simulink model "simulacion_tanques"  (R2018a)
settings: Solver=FixedStepAuto  StartTime=0.0  StopTime=4000  FixedStep=1  RelTol=1e-3
InitFcn:
  | parametros
values from neighbouring files (symbols this model uses):
  A = [A11 A12 A13 ; A21 A22 A23 ; A31 A32 A33 ]    [parametros.m]
  B = [B11 B12 ; B21 B22 ;B31 B32 ]    [parametros.m]
  C = eye(3)    [parametros.m]
  flow_rate_1_ptf = 0.35e-4    (= 3.5e-05)    [ini_para.m]    (also in parametros.m)
  flow_rate_2_ptf = 0.375e-4    (= 3.75e-05)    [ini_para.m]    (also in parametros.m)
  h_max = 0.62    [ini_para.m]    (also in parametros.m)
  h_min = 0    [ini_para.m]    (also in parametros.m)
  K1 = [21.6 3 -5;2.9 19 -4]*10e-4    [ini_para.m]    (also in parametros.m; uio_linear.m = K1')
  K2 = [-0.95 -0.32;-0.3 -0.91]*10e-4    [ini_para.m]    (also in parametros.m)
  level_1_ini = 0.4    [ini_para.m]    (also in parametros.m)
  level_1_ptf = 0.4    [ini_para.m]    (also in parametros.m)
  level_2_ini = 0.2    [ini_para.m]    (also in parametros.m)
  level_2_ptf = 0.2    [ini_para.m]    (also in parametros.m)
  level_3_ini = 0.3    [ini_para.m]    (also in parametros.m)
  level_3_ptf = 0.3    [ini_para.m]    (also in parametros.m)
  q_max = 1.5e-4    (= 0.00015)    [ini_para.m]    (also in parametros.m)
  q_min = 0    [ini_para.m]    (also in parametros.m)
  Te = 1    [ini_para.m]    (also in parametros.m)
undefined symbols (not defined in the file or in its folder): DiscIntNeverNeededParam
settings Model: Creator=cmparedes  LastModifiedBy=cmparedes

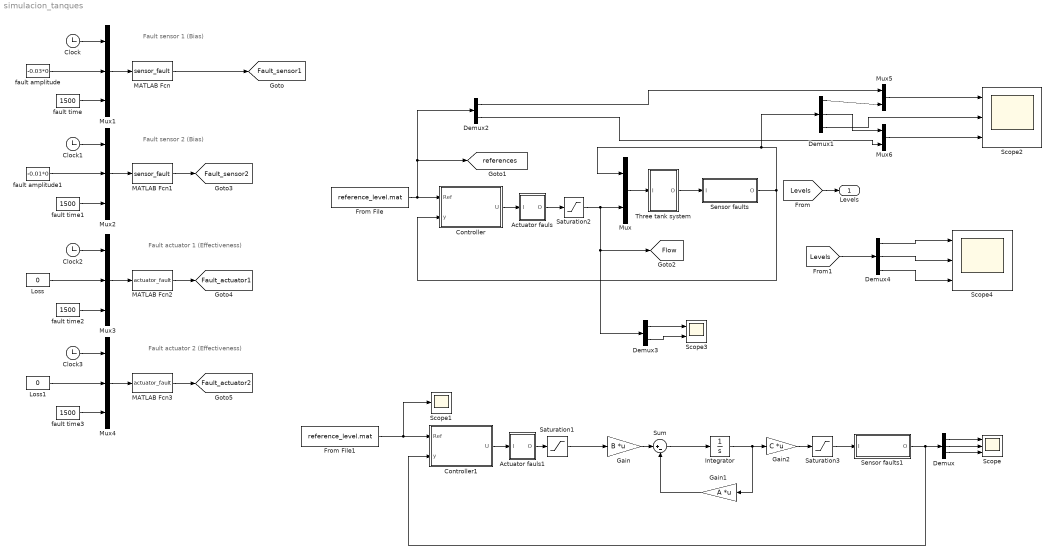
== system simulacion_tanques ==
  note: Fault actuator 2 (Effectiveness)
  note: Fault actuator 1 (Effectiveness)
  note: Fault sensor 1 (Bias)
  note: Fault sensor 2 (Bias)
  Actuator fauls : Subsystem
  Actuator fauls1 : Subsystem
  Clock{,1..3} (4 alike) : Clock
  Controller : Subsystem
  Controller1 : Subsystem
  Demux : Demux  Outputs=3
  Demux1 : Demux  Outputs=3
  Demux2 : Demux  Outputs=2
  Demux3 : Demux  Outputs=2
  Demux4 : Demux  Outputs=3
  From File : FromFile  FileName=reference_level.mat  SampleTime=1
  From File1 : FromFile  FileName=reference_level.mat  SampleTime=1
  Gain : Gain  Gain=B  Multiplication=Matrix(K*u)
  Gain1 : Gain  Gain=A  Multiplication=Matrix(K*u)
  Gain2 : Gain  Gain=C  Multiplication=Matrix(K*u)
  Integrator : Integrator  InitialCondition=[level_1_ini;level_3_ini;level_2_ini]
  Loss : Constant  Value=0
  Loss1 : Constant  Value=0
  MATLAB Fcn : MATLABFcn  MATLABFcn=sensor_fault
  MATLAB Fcn1 : MATLABFcn  MATLABFcn=sensor_fault
  MATLAB Fcn2 : MATLABFcn  MATLABFcn=actuator_fault
  MATLAB Fcn3 : MATLABFcn  MATLABFcn=actuator_fault
  Mux : Mux  Inputs=2
  Mux{1..4} (4 alike) : Mux  Inputs=3
  Mux5 : Mux  Inputs=2
  Mux6 : Mux  Inputs=2
  Saturation1 : Saturate  UpperLimit=q_max  LowerLimit=q_min
  Saturation2 : Saturate  UpperLimit=q_max  LowerLimit=q_min
  Saturation3 : Saturate  UpperLimit=h_max  LowerLimit=h_min
  Scope : Scope  NumInputPorts=3
  Scope1 : Scope
  Scope2 : Scope  NumInputPorts=3
  Scope3 : Scope  NumInputPorts=2
  Scope4 : Scope  NumInputPorts=3
  Sensor faults : Subsystem
  Sensor faults1 : Subsystem
  Sum : Sum  Inputs=|+-
  Three tank system : Subsystem
  fault amplitude : Constant  Value=-0.03*0
  fault amplitude1 : Constant  Value=-0.01*0
  fault time{,1..3} (4 alike) : Constant  Value=1500
  Levels : Outport
  tag scope: Fault_actuator1=global, Fault_actuator2=global, Fault_sensor1=global, Fault_sensor2=global, Flow=global, references=global
  wires:
  Three tank system/1(O) -> Sensor faults/1(I)
  [Levels] -> Levels/1
  Actuator fauls/1(O) -> Saturation2/1
  Sensor faults/1(O) -> Demux1/1, Mux/1, Controller/2(y)
  Saturation2/1 -> Mux/2, Demux3/1, [Flow]
  From File/1 -> Demux2/1, [references], Controller/1(Ref)
  Mux/1 -> Three tank system/1(I)
  Controller/1(U) -> Actuator fauls/1(I)
  Clock1/1 -> Mux2/1
  fault time1/1 -> Mux2/3
  Loss1/1 -> Mux4/2
  Clock/1 -> Mux1/1
  MATLAB Fcn3/1 -> [Fault_actuator2]
  fault time3/1 -> Mux4/3
  MATLAB Fcn2/1 -> [Fault_actuator1]
  Mux3/1 -> MATLAB Fcn2/1
  Clock3/1 -> Mux4/1
  fault amplitude/1 -> Mux1/2
  Mux2/1 -> MATLAB Fcn1/1
  MATLAB Fcn/1 -> [Fault_sensor1]
  Loss/1 -> Mux3/2
  MATLAB Fcn1/1 -> [Fault_sensor2]
  fault time/1 -> Mux1/3
  fault time2/1 -> Mux3/3
  Mux1/1 -> MATLAB Fcn/1
  Clock2/1 -> Mux3/1
  Mux4/1 -> MATLAB Fcn3/1
  fault amplitude1/1 -> Mux2/2
  Gain/1 -> Sum/1
  Sum/1 -> Integrator/1
  Gain1/1 -> Sum/2
  Integrator/1 -> Gain2/1, Gain1/1
  Gain2/1 -> Saturation3/1
  Sensor faults1/1(O) -> Demux/1, Controller1/2(y)
  Actuator fauls1/1(O) -> Saturation1/1
  Controller1/1(U) -> Actuator fauls1/1(I)
  Saturation1/1 -> Gain/1
  From File1/1 -> Scope1/1, Controller1/1(Ref)
  Saturation3/1 -> Sensor faults1/1(I)
  Demux/1 -> Scope/1
  Demux/2 -> Scope/2
  Demux/3 -> Scope/3
  Demux1/1 -> Mux5/2
  Demux2/1 -> Mux5/1
  Mux5/1 -> Scope2/1
  Demux2/2 -> Mux6/2
  Mux6/1 -> Scope2/3
  Demux1/2 -> Mux6/1
  Demux1/3 -> Scope2/2
  Demux3/1 -> Scope3/1
  Demux3/2 -> Scope3/2
  [Levels] -> Demux4/1
  Demux4/1 -> Scope4/1
  Demux4/2 -> Scope4/2
  Demux4/3 -> Scope4/3

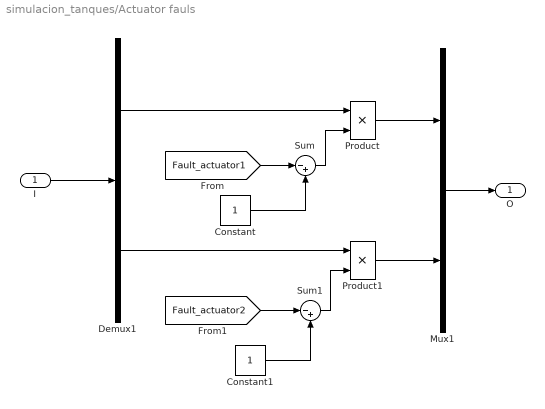
== system simulacion_tanques/Actuator fauls ==
  I : Inport
  Constant : Constant
  Constant1 : Constant
  Demux1 : Demux  Outputs=2
  Mux1 : Mux  Inputs=2
  Product : Product  SaturateOnIntegerOverflow=on  OutDataTypeStr=Inherit: Same as first input
  Product1 : Product  SaturateOnIntegerOverflow=on  OutDataTypeStr=Inherit: Same as first input
  Sum : Sum  Inputs=|-+  SaturateOnIntegerOverflow=on
  Sum1 : Sum  Inputs=|-+  SaturateOnIntegerOverflow=on
  O : Outport
  wires:
  Product1/1 -> Mux1/2
  Demux1/2 -> Product1/1
  Product/1 -> Mux1/1
  Demux1/1 -> Product/1
  Mux1/1 -> O/1
  I/1 -> Demux1/1
  [Fault_actuator1] -> Sum/1
  Constant/1 -> Sum/2
  Sum/1 -> Product/2
  [Fault_actuator2] -> Sum1/1
  Sum1/1 -> Product1/2
  Constant1/1 -> Sum1/2

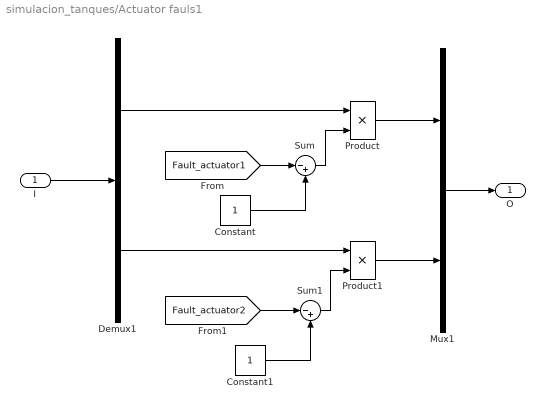
== system simulacion_tanques/Actuator fauls1 ==
  I : Inport
  Constant : Constant
  Constant1 : Constant
  Demux1 : Demux  Outputs=2
  Mux1 : Mux  Inputs=2
  Product : Product  SaturateOnIntegerOverflow=on  OutDataTypeStr=Inherit: Same as first input
  Product1 : Product  SaturateOnIntegerOverflow=on  OutDataTypeStr=Inherit: Same as first input
  Sum : Sum  Inputs=|-+  SaturateOnIntegerOverflow=on
  Sum1 : Sum  Inputs=|-+  SaturateOnIntegerOverflow=on
  O : Outport
  wires:
  Product1/1 -> Mux1/2
  Demux1/2 -> Product1/1
  Product/1 -> Mux1/1
  Demux1/1 -> Product/1
  Mux1/1 -> O/1
  I/1 -> Demux1/1
  [Fault_actuator1] -> Sum/1
  Constant/1 -> Sum/2
  Sum/1 -> Product/2
  [Fault_actuator2] -> Sum1/1
  Sum1/1 -> Product1/2
  Constant1/1 -> Sum1/2

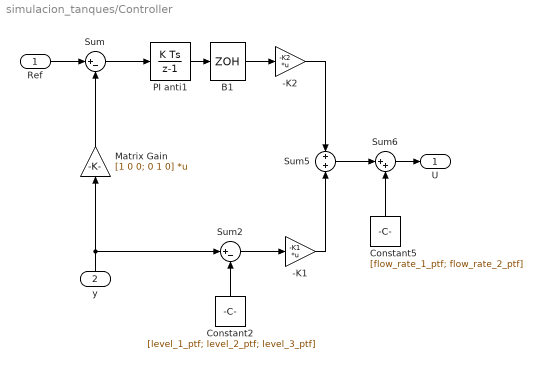
== system simulacion_tanques/Controller ==
  Ref : Inport
  y : Inport  Port=2
  -K1 : Gain  Gain=-K1  Multiplication=Matrix(K*u)  SaturateOnIntegerOverflow=on  OutDataTypeStr=Inherit: Same as input  ParamDataTypeStr=Inherit: Same as input
  -K2 : Gain  Gain=-K2  Multiplication=Matrix(K*u)  SaturateOnIntegerOverflow=on  OutDataTypeStr=Inherit: Same as input  ParamDataTypeStr=Inherit: Same as input
  B1 : ZeroOrderHold  SampleTime=Te
  Constant2 : Constant  Value=[level_1_ptf; level_2_ptf; level_3_ptf]
  Constant5 : Constant  Value=[flow_rate_1_ptf; flow_rate_2_ptf]
  Matrix Gain : Gain  Gain=[1 0 0; 0 1 0]  Multiplication=Matrix(K*u)  SaturateOnIntegerOverflow=on  OutDataTypeStr=Inherit: Same as input  ParamDataTypeStr=Inherit: Same as input
  PI anti1 : DiscreteIntegrator  SampleTime=Te  LimitOutput=on  UpperSaturationLimit=100  LowerSaturationLimit=-100  ICPrevOutput=DiscIntNeverNeededParam  ICPrevScaledInput=DiscIntNeverNeededParam
  Sum : Sum  Inputs=|+-  SaturateOnIntegerOverflow=on  InputSameDT=on  OutDataTypeStr=Inherit: Same as first input
  Sum2 : Sum  Inputs=|+-  SaturateOnIntegerOverflow=on  InputSameDT=on  OutDataTypeStr=Inherit: Same as first input
  Sum5 : Sum  SaturateOnIntegerOverflow=on  InputSameDT=on  OutDataTypeStr=Inherit: Same as first input
  Sum6 : Sum  Inputs=|++  SaturateOnIntegerOverflow=on  InputSameDT=on  OutDataTypeStr=Inherit: Same as first input
  U : Outport
  wires:
  Constant2/1 -> Sum2/2
  Sum2/1 -> -K1/1
  Sum/1 -> PI anti1/1
  -K2/1 -> Sum5/1
  -K1/1 -> Sum5/2
  Sum5/1 -> Sum6/1
  Constant5/1 -> Sum6/2
  PI anti1/1 -> B1/1
  B1/1 -> -K2/1
  Matrix Gain/1 -> Sum/2
  Ref/1 -> Sum/1
  y/1 -> Sum2/1, Matrix Gain/1
  Sum6/1 -> U/1

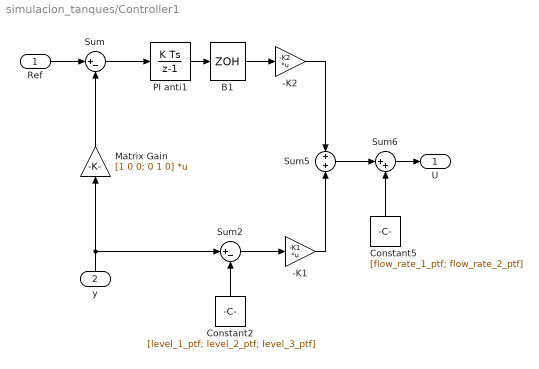
== system simulacion_tanques/Controller1 ==
  Ref : Inport
  y : Inport  Port=2
  -K1 : Gain  Gain=-K1  Multiplication=Matrix(K*u)  SaturateOnIntegerOverflow=on  OutDataTypeStr=Inherit: Same as input  ParamDataTypeStr=Inherit: Same as input
  -K2 : Gain  Gain=-K2  Multiplication=Matrix(K*u)  SaturateOnIntegerOverflow=on  OutDataTypeStr=Inherit: Same as input  ParamDataTypeStr=Inherit: Same as input
  B1 : ZeroOrderHold
  Constant2 : Constant  Value=[level_1_ptf; level_2_ptf; level_3_ptf]
  Constant5 : Constant  Value=[flow_rate_1_ptf; flow_rate_2_ptf]
  Matrix Gain : Gain  Gain=[1 0 0; 0 1 0]  Multiplication=Matrix(K*u)  SaturateOnIntegerOverflow=on  OutDataTypeStr=Inherit: Same as input  ParamDataTypeStr=Inherit: Same as input
  PI anti1 : DiscreteIntegrator  LimitOutput=on  UpperSaturationLimit=100  LowerSaturationLimit=-100  ICPrevOutput=DiscIntNeverNeededParam  ICPrevScaledInput=DiscIntNeverNeededParam
  Sum : Sum  Inputs=|+-  SaturateOnIntegerOverflow=on  InputSameDT=on  OutDataTypeStr=Inherit: Same as first input
  Sum2 : Sum  Inputs=|+-  SaturateOnIntegerOverflow=on  InputSameDT=on  OutDataTypeStr=Inherit: Same as first input
  Sum5 : Sum  SaturateOnIntegerOverflow=on  InputSameDT=on  OutDataTypeStr=Inherit: Same as first input
  Sum6 : Sum  Inputs=|++  SaturateOnIntegerOverflow=on  InputSameDT=on  OutDataTypeStr=Inherit: Same as first input
  U : Outport
  wires:
  Constant2/1 -> Sum2/2
  Sum2/1 -> -K1/1
  Sum/1 -> PI anti1/1
  -K2/1 -> Sum5/1
  -K1/1 -> Sum5/2
  Sum5/1 -> Sum6/1
  Constant5/1 -> Sum6/2
  PI anti1/1 -> B1/1
  B1/1 -> -K2/1
  Matrix Gain/1 -> Sum/2
  Ref/1 -> Sum/1
  y/1 -> Sum2/1, Matrix Gain/1
  Sum6/1 -> U/1

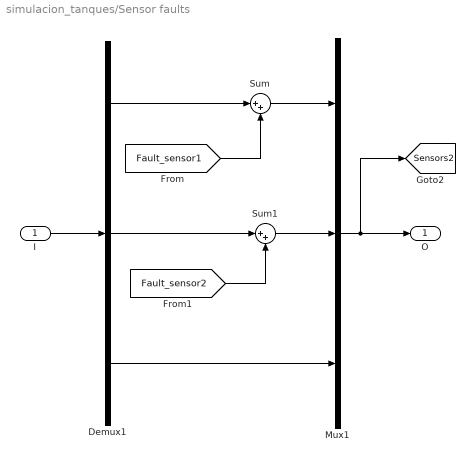
== system simulacion_tanques/Sensor faults ==
  I : Inport
  Demux1 : Demux  Outputs=3
  Mux1 : Mux  Inputs=3
  Sum : Sum  Inputs=|++  SaturateOnIntegerOverflow=on
  Sum1 : Sum  Inputs=|++  SaturateOnIntegerOverflow=on
  O : Outport
  tag scope: Sensors2=global
  wires:
  I/1 -> Demux1/1
  Mux1/1 -> O/1, [Sensors2]
  Demux1/1 -> Sum/1
  Sum/1 -> Mux1/1
  [Fault_sensor1] -> Sum/2
  [Fault_sensor2] -> Sum1/2
  Demux1/3 -> Mux1/3
  Demux1/2 -> Sum1/1
  Sum1/1 -> Mux1/2

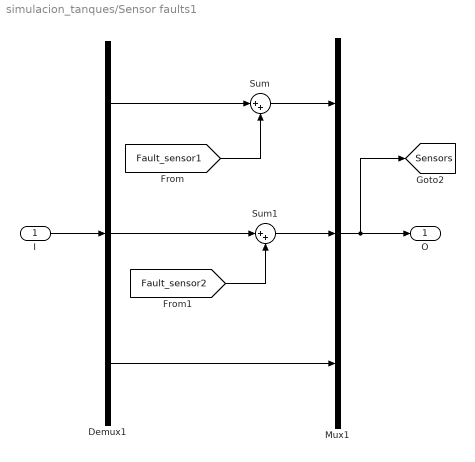
== system simulacion_tanques/Sensor faults1 ==
  I : Inport
  Demux1 : Demux  Outputs=3
  Mux1 : Mux  Inputs=3
  Sum : Sum  Inputs=|++  SaturateOnIntegerOverflow=on
  Sum1 : Sum  Inputs=|++  SaturateOnIntegerOverflow=on
  O : Outport
  tag scope: Sensors=global
  wires:
  I/1 -> Demux1/1
  Mux1/1 -> O/1, [Sensors]
  Demux1/1 -> Sum/1
  Sum/1 -> Mux1/1
  [Fault_sensor1] -> Sum/2
  [Fault_sensor2] -> Sum1/2
  Demux1/3 -> Mux1/3
  Demux1/2 -> Sum1/1
  Sum1/1 -> Mux1/2

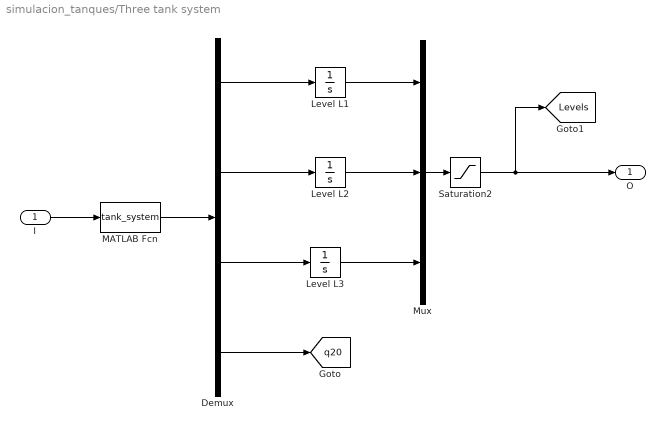
== system simulacion_tanques/Three tank system ==
  I : Inport
  Demux : Demux
  Level L1 : Integrator  InitialCondition=level_1_ini
  Level L2 : Integrator  InitialCondition=level_2_ini
  Level L3 : Integrator  InitialCondition=level_3_ini
  MATLAB Fcn : MATLABFcn  MATLABFcn=tank_system  OutputDimensions=4
  Mux : Mux  Inputs=3
  Saturation2 : Saturate  UpperLimit=h_max  LowerLimit=h_min
  O : Outport
  tag scope: Levels=global, q20=global
  wires:
  I/1 -> MATLAB Fcn/1
  MATLAB Fcn/1 -> Demux/1
  Demux/1 -> Level L1/1
  Demux/2 -> Level L2/1
  Demux/3 -> Level L3/1
  Level L2/1 -> Mux/2
  Level L3/1 -> Mux/3
  Mux/1 -> Saturation2/1
  Demux/4 -> [q20]
  Level L1/1 -> Mux/1
  Saturation2/1 -> [Levels], O/1
